simulink model "PROJET_IO"  (R2020a)
settings: Solver=ode4  StartTime=0.0  StopTime=StopTime  FixedStep=Te  RelTol=1e-3
values from neighbouring files (symbols this model uses):
  Te = 0.025    [PROJET.m]    (also in exitation_de_systeme.m; save_STEP.mat)
undefined symbols (not defined in the file or in its folder): National_Instruments, PCI
libraries: sldrtlib x2
settings Model: Creator=lespiaucq  LastModifiedBy=lespiaucq
settings RTWCC: Description=Simulink Desktop Real-Time  SystemTargetFile=sldrt.tlc  TemplateMakefile=sldrt.tmf  RTWCompilerOptimization=on
settings CodeAppCC: MaxIdLength=95
settings SimulinkDesktopRealTimeCC: TargetPreCompLibLocation=C:\Program Files\MATLAB\R2020a\toolbox\sldrt\lib\win64

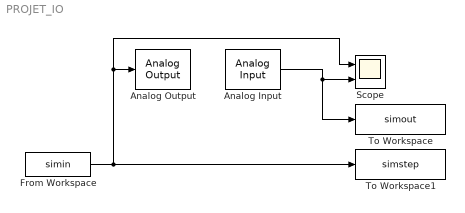
== system PROJET_IO ==
  Analog Input : sldrtlib/Analog Input  SampleTime=Te  MaxMissedTicks=10  ShowMissedTicks=off  YieldWhenWaiting=off  DrvName=National_Instruments/PCI-6024E  DrvAddress=4294967295  DrvOptions=[0 0 0 0 0 0]  Channels=1  RangeMode=1  VoltRange=1  DataType=1
      settings: AttributesFormatString=National Instruments\nPCI-6024E [auto]
  Analog Output : sldrtlib/Analog Output  SampleTime=Te  MaxMissedTicks=10  ShowMissedTicks=off  YieldWhenWaiting=off  DrvName=National_Instruments/PCI-6024E  DrvAddress=4294967295  DrvOptions=[0 0 0 0 0 0]  Channels=1  RangeMode=1  VoltRange=1  InitialValue=[]  FinalValue=[]
      settings: AttributesFormatString=National Instruments\nPCI-6024E [auto]
  From Workspace : FromWorkspace  VariableName=simin
  Scope : Scope  NumInputPorts=2
  To Workspace : ToWorkspace  VariableName=simout  SaveFormat=Timeseries  SampleTime=-1
  To Workspace1 : ToWorkspace  VariableName=simstep  SaveFormat=Timeseries  SampleTime=-1
  wires:
  Analog Input/1 -> To Workspace/1, Scope/2
  From Workspace/1 -> To Workspace1/1, Analog Output/1, Scope/1
